simulink model "fb_lin"  (R2022b)
settings: Solver=ode45  StartTime=0.0  StopTime=20  RelTol=1e-6
values from neighbouring files (symbols this model uses):
  delta1 = 1/10    (= 0.1)    [main.m]
  delta2 = 1/5    (= 0.2)    [main.m]
  K = place(Az,B,[-3 -4 -5 -6])    [main.m]
  k1 = 2/5    (= 0.4)    [main.m]
  k2 = 1    [main.m]
  m1 = 1    [main.m]
  m2 = 2    [main.m]
  miu1 = 1/6    (= 0.166666666667)    [main.m]
  miu2 = 1/10    (= 0.1)    [main.m]
settings Model: Creator=Alex  LastModifiedBy=Alex

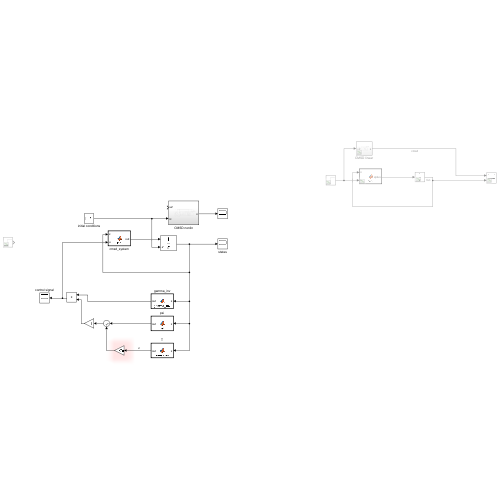
[thumbnail: Simulink's stored preview of the top-level diagram]
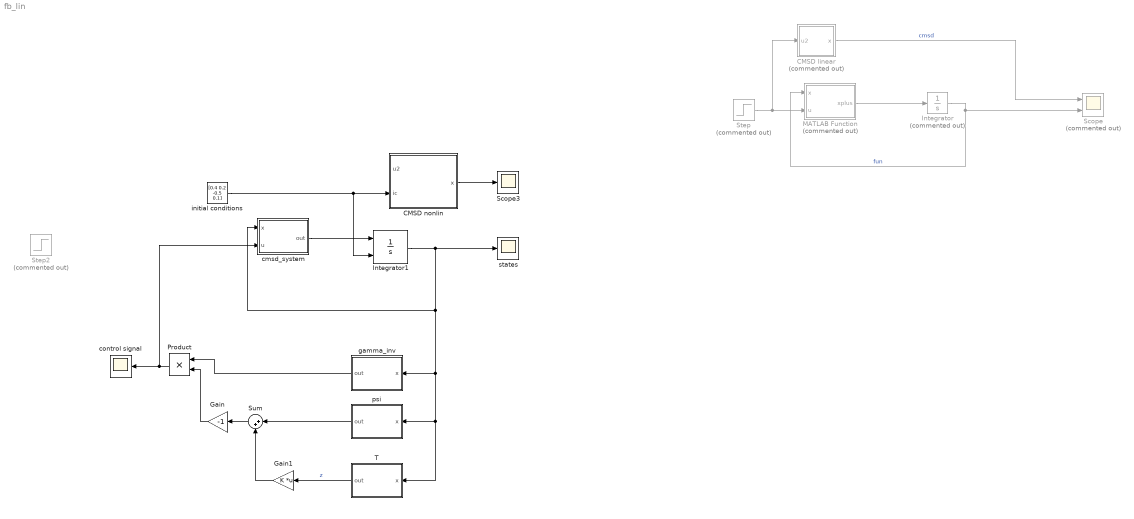
== system fb_lin ==
  CMSD linear : Subsystem  Commented=on
  CMSD nonlin : Subsystem
  Gain : Gain  Gain=-1
  Gain1 : Gain  Gain=K  Multiplication=Matrix(K*u)
  Integrator : Integrator  Commented=on  InitialCondition=[0 0 0 0]'
  Integrator1 : Integrator  InitialConditionSource=external  InitialCondition=[0.1 0.02 -0.1 -0.1]'
  MATLAB Function : MATLAB Function  Commented=on  TreatAsAtomicUnit=on
  Product : Product
  Scope : Scope  Commented=on  NumInputPorts=2
  Scope3 : Scope
  Step : Step  Commented=on  Time=0  SampleTime=0
  Step2 : Step  Commented=on  Time=0  After=0.1  SampleTime=0
  Sum : Sum  Inputs=|++
  T : MATLAB Function  TreatAsAtomicUnit=on
  cmsd_system : MATLAB Function  TreatAsAtomicUnit=on
  control signal : Scope
  gamma_inv : MATLAB Function  TreatAsAtomicUnit=on
  initial conditions : Constant  Value=[0.4 0.2 -0.5 0.1]
  psi : MATLAB Function  TreatAsAtomicUnit=on
  states : Scope
  wires:
  MATLAB Function/1(xplus) -> Integrator/1
  Step/1 -> CMSD linear/1(u2), MATLAB Function/2(u)
  Integrator/1 -> Scope/2, MATLAB Function/1(x)  "fun"
  CMSD linear/1(x) -> Scope/1  "cmsd"
  cmsd_system/1(out) -> Integrator1/1
  Integrator1/1 -> psi/1(x), T/1(x), gamma_inv/1(x), cmsd_system/1(x), states/1
  gamma_inv/1(out) -> Product/1
  psi/1(out) -> Sum/1
  Sum/1 -> Gain/1
  T/1(out) -> Gain1/1  "z"
  Gain/1 -> Product/2
  Product/1 -> control signal/1, cmsd_system/2(u)
  Gain1/1 -> Sum/2
  initial conditions/1 -> CMSD nonlin/2(ic), Integrator1/2
  CMSD nonlin/1(x) -> Scope3/1

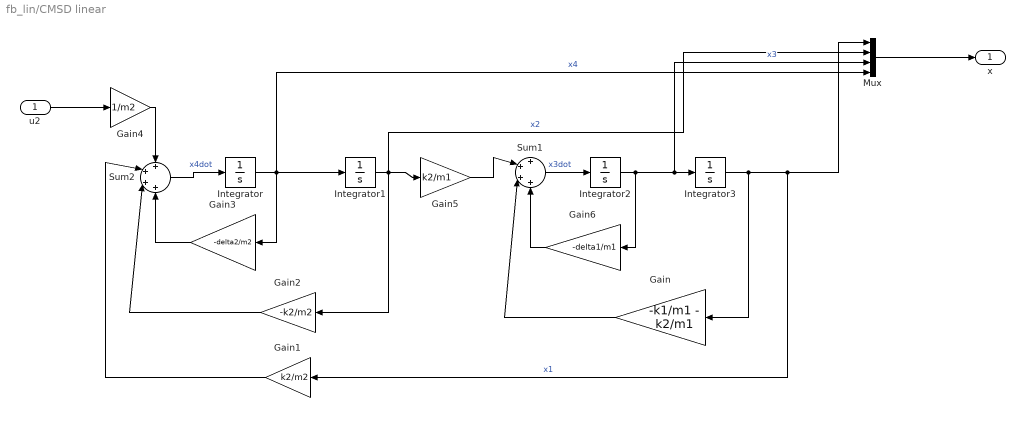
== system fb_lin/CMSD linear ==
  u2 : Inport
  Gain : Gain  Gain=-k1/m1 - k2/m1
  Gain1 : Gain  Gain=k2/m2
  Gain2 : Gain  Gain=-k2/m2
  Gain3 : Gain  Gain=-delta2/m2
  Gain4 : Gain  Gain=1/m2
  Gain5 : Gain  Gain=k2/m1
  Gain6 : Gain  Gain=-delta1/m1
  Integrator{,1..3} (4 alike) : Integrator
  Mux : Mux
  Sum1 : Sum  Inputs=++++
  Sum2 : Sum  Inputs=++++
  x : Outport
  wires:
  Integrator1/1 -> Mux/2, Gain2/1, Gain5/1  "x2"
  Gain6/1 -> Sum1/4
  Gain/1 -> Sum1/3
  u2/1 -> Gain4/1
  Integrator3/1 -> Gain/1, Mux/1, Gain1/1  "x1"
  Integrator/1 -> Mux/4, Gain3/1, Integrator1/1  "x4"
  Gain5/1 -> Sum1/2
  Gain4/1 -> Sum2/1
  Sum2/1 -> Integrator/1  "x4dot"
  Sum1/1 -> Integrator2/1  "x3dot"
  Integrator2/1 -> Gain6/1, Mux/3, Integrator3/1  "x3"
  Gain2/1 -> Sum2/3
  Gain1/1 -> Sum2/2
  Gain3/1 -> Sum2/4
  Mux/1 -> x/1

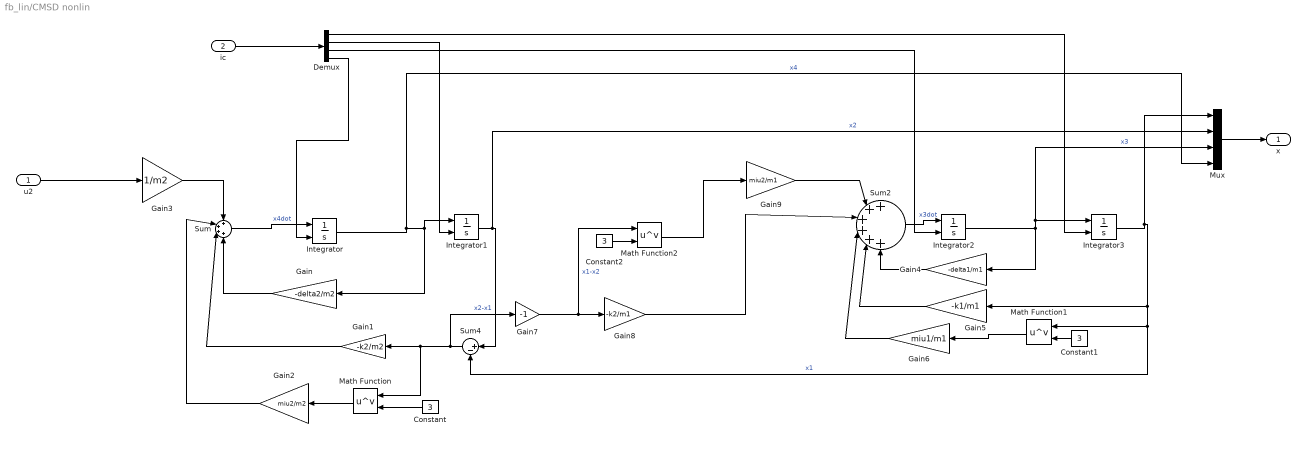
== system fb_lin/CMSD nonlin ==
  u2 : Inport
  ic : Inport  Port=2
  Constant : Constant  Value=3
  Constant1 : Constant  Value=3
  Constant2 : Constant  Value=3
  Demux : Demux
  Gain : Gain  Gain=-delta2/m2
  Gain1 : Gain  Gain=-k2/m2
  Gain2 : Gain  Gain=miu2/m2
  Gain3 : Gain  Gain=1/m2
  Gain4 : Gain  Gain=-delta1/m1
  Gain5 : Gain  Gain=-k1/m1
  Gain6 : Gain  Gain=miu1/m1
  Gain7 : Gain  Gain=-1
  Gain8 : Gain  Gain=-k2/m1
  Gain9 : Gain  Gain=miu2/m1
  Integrator{,1..3} (4 alike) : Integrator  InitialConditionSource=external
  Math Function : Math  Operator=pow
  Math Function1 : Math  Operator=pow
  Math Function2 : Math  Operator=pow
  Mux : Mux
  Sum : Sum  Inputs=++++
  Sum2 : Sum  Inputs=++++++
  Sum4 : Sum  Inputs=|+-
  x : Outport
  wires:
  Gain4/1 -> Sum2/6
  Integrator/1 -> Mux/4, Gain/1, Integrator1/1  "x4"
  Sum4/1 -> Gain7/1, Math Function/1, Gain1/1  "x2-x1"
  Integrator3/1 -> Mux/1, Sum4/2, Math Function1/1, Gain5/1  "x1"
  Gain8/1 -> Sum2/3
  Gain7/1 -> Math Function2/1, Gain8/1  "x1-x2"
  Math Function2/1 -> Gain9/1
  Gain3/1 -> Sum/1
  Gain5/1 -> Sum2/5
  Gain1/1 -> Sum/3
  Constant2/1 -> Math Function2/2
  Gain9/1 -> Sum2/2
  Sum/1 -> Integrator/1  "x4dot"
  Math Function1/1 -> Gain6/1
  Gain/1 -> Sum/4
  Gain2/1 -> Sum/2
  Integrator1/1 -> Mux/2, Sum4/1  "x2"
  Constant/1 -> Math Function/2
  Math Function/1 -> Gain2/1
  Integrator2/1 -> Mux/3, Integrator3/1, Gain4/1  "x3"
  Gain6/1 -> Sum2/4
  u2/1 -> Gain3/1
  Sum2/1 -> Integrator2/1  "x3dot"
  Constant1/1 -> Math Function1/2
  Mux/1 -> x/1
  ic/1 -> Demux/1
  Demux/4 -> Integrator/2
  Demux/3 -> Integrator2/2
  Demux/2 -> Integrator1/2
  Demux/1 -> Integrator3/2

== matlab function fb_lin/MATLAB Function ==
  data: x input; xplus output; u input
function xplus = fcn(x,u)

k1=2/5; % N/m
k2=1;
m1=1; % kg
m2=2;
delta1=1/10; %
delta2=1/5;
miu1=1/6; %
miu2=1/10;

A=[0 0 1 0;
   0 0 0 1;
   -k1/m1-k2/m1 , k2/m1 , -delta1/m1 , 0;
   k2/m2, -k2/m2 , 0 , -delta2/m2];

B=[0;
   0;
   0;
   1/m2];

xplus=A*x+B*u;

== matlab function fb_lin/gamma_inv ==
  data: x input; out output
function out= gamma_inv(x)

k1=2/5; % N/m
k2=1;
m1=1; % kg
m2=2;
delta1=1/10; %Ns/m
delta2=1/5;
miu1=1/6; %
miu2=1/10;


out=m2/(k2-3*miu2*(x(1)-x(2)).^2);

== matlab function fb_lin/psi ==
  data: x input; out output
function out= psi(x)

k1=2/5; % N/m
k2=1;
m1=1; % kg
m2=2;
delta1=1/10; %
delta2=1/5;
miu1=1/6; %
miu2=1/10;


x1=x(1);
x2=x(2);
x3=x(3);
x4=x(4);

x3dot=-delta1/m1*x3-k1/m1*x1+miu1/m1*x1.^3-k2/m1*(x1-x2)+miu2/m1*(x1-x2).^3;

psi=x3dot*(3*miu1*x1.^2+3*miu2*(x1-x2).^2)+6*miu1*x1.*x3.^2+6*miu2*x3.*(x1-x2).*(x3-x4).^2+...
    (k2-3*miu2*(x1-x2).^2)/m2.*(-delta2*x4-k2*x2+miu2*(x2-x1).^3)-3*k2*miu2/m2*x1.*(x1-x2).^2;
out=psi;

== matlab function fb_lin/T ==
  data: x input; out output
function out= transform(x)

k1=2/5; % N/m
k2=1;
m1=1; % kg
m2=2;
delta1=1/10; %Ns/m
delta2=1/5;
miu1=1/6; %
miu2=1/10;


z=zeros(4,1);
x1=x(1);
x2=x(2);
x3=x(3);
x4=x(4);

z(1)=x1;
z(2)=x3;
z(3)=-delta1/m1*x3-k1/m1*x1+miu1/m1*x1.^3-k2/m1*(x1-x2)+miu2/m1*(x1-x2).^3;
z(4)=x3*(-k1/m1+3*miu1/m1*x1.^2-k2/m1+3*miu2/m1*(x1-x2).^2)+...
    x4*(k2/m1-3*miu2/m1*(x1-x2).^2)-delta1/m1*z(3);
out=z;

== matlab function fb_lin/cmsd_system ==
  data: x input; u input; out output
function out = fcn(x,u)

k1=2/5; % N/m
k2=1;
m1=1; % kg
m2=2;
delta1=1/10; %Ns/m
delta2=1/5;
miu1=1/6; %
miu2=1/10;
g=[0 0 0 1/m2]';

xdot=[x(3);...
      x(4);...
      -delta1/m1*x(3)-k1/m1*x(1)+miu1/m1 * x(1)^3 - k2/m1 * (x(1)-x(2))+miu2/m1*(x(1)-x(2))^3;...
      -delta2/m2*x(4)-k2/m2*(x(2)-x(1))+miu2/m2*(x(2)-x(1))^3];



out= xdot+g*u;
